simulink model "SCR_Buck_CL_17a"  (R2017b)
settings: Solver=FixedStepAuto  StartTime=0.0  StopTime=0.5  FixedStep=1e-6  MaxStep=1e-4  RelTol=1e-3
undefined symbols (not defined in the file): C
libraries: powerlib x16, simulink x5
settings Model: Creator=Suman Maiti  LastModifiedBy=Shuvam
settings DataIOCC: SaveFormat=StructureWithTime
settings OptimizationCC: LifeSpan=inf
settings DebuggingCC: AlgebraicLoopMsg=none  ArtificialAlgebraicLoopMsg=none  SFExecutionAtInitializationDiag=none
settings HardwareCC: ProdBitPerSizeT=32  ProdBitPerPtrDiffT=32  ProdWordSize=32  ProdHWDeviceType=Specified
settings CodeAppCC: StateflowObjectComments=on
settings SimscapeCC: SimscapeNormalizeSystem=off

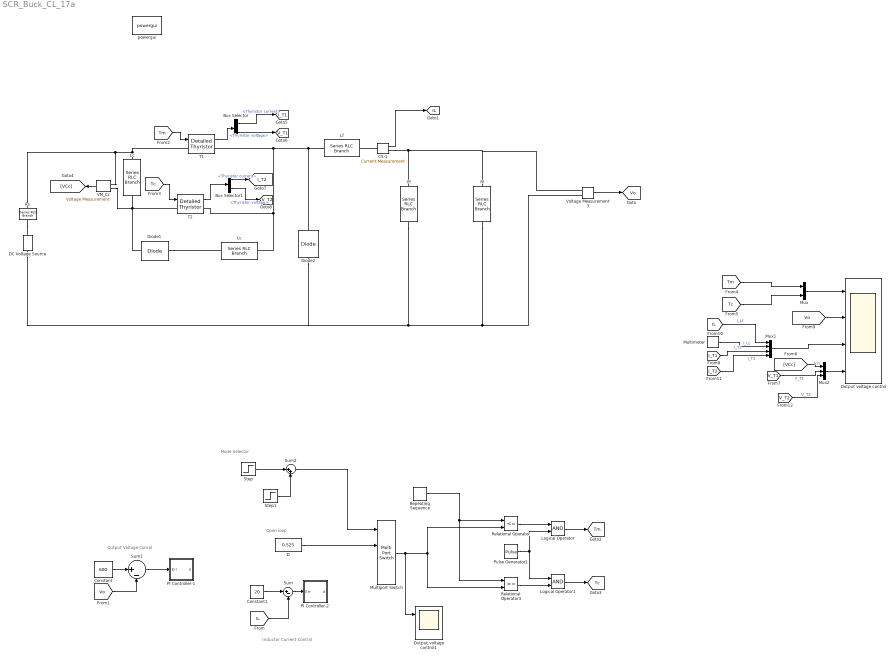
== system SCR_Buck_CL_17a ==
  note: Mode Selector
  note: Inductor Current Control
  note: Open loop
  note: Output Voltage Conrol
  Bus Selector : BusSelector  OutputSignals=Thyristor current,Thyristor voltage
  Bus Selector1 : BusSelector  OutputSignals=Thyristor current,Thyristor voltage
  CS-1 : powerlib/Measurements/Current Measurement  PhasorSimulation=off  OutputType=Complex  PSBequivalent=0
  Cc : powerlib/Elements/Series RLC Branch  LConnTagsString=__new0  RConnTagsString=__new0  BranchType=C  Resistance=0.00000001  Inductance=50e-3  SetiL0=off  InitialCurrent=0  Capacitance=0.2e-6  Setx0=on  InitialVoltage=1000  Measurements=None
  Cf : powerlib/Elements/Series RLC Branch  LConnTagsString=__new0  RConnTagsString=__new0  BranchType=C  Resistance=1  Inductance=15e-3  SetiL0=off  InitialCurrent=0  Capacitance=330e-6  Setx0=on  InitialVoltage=600  Measurements=None
  Constant : Constant  Value=600
  Constant1 : Constant  Value=20
  D : Constant  Value=0.525
  DC Voltage Source : powerlib/Electrical Sources/DC Voltage Source  Amplitude=1000  Measurements=None
  Diode1 : powerlib/Power Electronics/Diode  Ron=0.001  Lon=0  Vf=0  IC=0  UseSnubber=0  Rs=500  Cs=2e-9  Measurements=off
  Diode2 : powerlib/Power Electronics/Diode  Ron=0.001  Lon=0  Vf=0  IC=0  UseSnubber=0  Rs=500000  Cs=250e-9  Measurements=off
  Lc : powerlib/Elements/Series RLC Branch  LConnTagsString=__new0  RConnTagsString=__new0  BranchType=L  Resistance=1  Inductance=0.25e-3  SetiL0=off  InitialCurrent=0  Capacitance=C  Setx0=on  InitialVoltage=Vc  Measurements=Branch current
  Lf : powerlib/Elements/Series RLC Branch  LConnTagsString=__new0  RConnTagsString=__new0  BranchType=L  Resistance=1  Inductance=24e-3  SetiL0=off  InitialCurrent=0  Capacitance=C  Setx0=on  InitialVoltage=Vc  Measurements=None
  Logical Operator : Logic  AllPortsSameDT=off  OutDataTypeStr=boolean
  Logical Operator1 : Logic  AllPortsSameDT=off  OutDataTypeStr=boolean
  Multimeter : powerlib/Measurements/Multimeter  PhasorSimulation=off  OutputType=Complex  sel=1  L=1  Gain=1  yselected={'Ib: Lc'};  PSBOutputType=1  PSBequivalent=0  AxesSetting=[0,0.1,-100,100]  Display=0  SavedBlockNames=-11
  Multiport Switch : MultiPortSwitch  DataPortOrder=Zero-based contiguous
  Mux : Mux  Inputs=2
  Mux1 : Mux
  Mux2 : Mux  Inputs=3
  Output voltage control : Scope  NumInputPorts=4
  Output voltage control1 : Scope  NumInputPorts=2
  PI Controller-1 : Subsystem
  PI Controller-2 : Subsystem
  Pulse Generator1 : DiscretePulseGenerator  PulseType=Time based  Period=1/10000  PulseWidth=50
  Relational Operator : RelationalOperator  Operator=<=  OutDataTypeStr=boolean  RndMeth=Simplest
  Relational Operator3 : RelationalOperator  OutDataTypeStr=boolean  RndMeth=Simplest
  Repeating Sequence : simulink/Sources/Repeating Sequence  rep_seq_t=[0 0.002]  rep_seq_y=[0 1]
  Rl : powerlib/Elements/Series RLC Branch  LConnTagsString=__new0  RConnTagsString=__new0  BranchType=R  Resistance=30  Inductance=15e-3  SetiL0=off  InitialCurrent=0  Capacitance=330e-6  Setx0=on  InitialVoltage=Vc  Measurements=None
  Rs : powerlib/Elements/Series RLC Branch  LConnTagsString=__new0  RConnTagsString=__new0  BranchType=R  Resistance=0.00000001  Inductance=50e-3  SetiL0=off  InitialCurrent=0  Capacitance=4.7e-6  Setx0=on  InitialVoltage=200  Measurements=None
  Step : Step  SampleTime=0
  Step1 : Step  Time=2  SampleTime=0
  Sum : Sum  Inputs=|+-
  Sum1 : Sum  Inputs=|+-
  Sum2 : Sum  Inputs=|++
  T1 : powerlib/Power Electronics/Detailed Thyristor  Ron=0.000001  Lon=1e-6  Vf=0  IL=0.1  Tq=30e-6  IC=0  Rs=inf  Cs=0  Measurements=on
      settings: SourceProductName=Simscape Power Systems  SourceProductBaseCode=PS
  T2 : powerlib/Power Electronics/Detailed Thyristor  Ron=0.000001  Lon=1e-6  Vf=0  IL=0.1  Tq=30e-6  IC=0  Rs=inf  Cs=0  Measurements=on
      settings: SourceProductName=Simscape Power Systems  SourceProductBaseCode=PS
  VM_Cc : powerlib/Measurements/Voltage Measurement  PhasorSimulation=off  OutputType=Complex  PSBequivalent=0
  Voltage Measurement3 : powerlib/Measurements/Voltage Measurement  PhasorSimulation=off  OutputType=Complex  PSBequivalent=0
  powergui : powerlib/powergui  Priority=1  SimulationMode=Discrete  SampleTime=1e-6  frequency=60  Iterations=50  frequencyindice=0  Pbase=100e6  ErrMax=1e-4  UnitsV=kV  UnitsW=MW  buscounter=0  FunctionMessages=off  echomessages=off  EnableUseOfTLC=off  CurrentSourceSwitches=off  DisableSnubberDevices=off  DisableRonSwitches=off  DisableVfSwitches=off  DisplayEquations=off  SolverType=Tustin/Backward Euler (TBE)  Interpol=off  ExternalGateDelay=off  methode=off  Ts=100  x0status=blocks  SPID=off  SwTol=0  HookPort=off  RestoreLinks=warning  ResistiveCurrentMeasurement=off  Frange=[0:2:500]  Ylog=off  Xlog=on  ShowGrid=off  save=off  variable=ZData  structure=ScopeData1  ZoomFFT=off  StartTime=1.45  cycles=2  DisplayStyle=1  fundamental=50  FreqAxis=off  MaxFrequency=2000  frequencyindicesteady=1  RmsSteady=1  display=off
  tag scope: IL=global, I_T1=global, I_T2=global, Tc=global, Tm=global, V_T1=global, V_T2=global, Vo=global
  wires:
  Voltage Measurement3/1 -> [Vo]
  [Tc] -> T2/1
  CS-1/1 -> [IL]
  [Tm] -> T1/1
  [IL] -> Sum/2
  Relational Operator/1 -> Logical Operator/1
  Pulse Generator1/1 -> Logical Operator1/1, Logical Operator/2
  Repeating Sequence/1 -> Relational Operator/1, Relational Operator3/1
  Relational Operator3/1 -> Logical Operator1/2
  Logical Operator/1 -> [Tm]
  Logical Operator1/1 -> [Tc]
  [Vo] -> Sum1/2
  Constant/1 -> Sum1/1
  Sum/1 -> PI Controller-2/1(Err)
  Constant1/1 -> Sum/1
  Step/1 -> Sum2/1
  Step1/1 -> Sum2/2
  Sum2/1 -> Multiport Switch/1
  [Vo] -> Output voltage control/2
  Mux1/1 -> Output voltage control/3
  Mux/1 -> Output voltage control/1
  [Tm] -> Mux/1
  [Tc] -> Mux/2
  [VCc] -> Mux2/1  "Vcc"
  VM_Cc/1 -> [VCc]
  Sum1/1 -> PI Controller-1/1(Err)
  Multimeter/1 -> Mux1/2  "I_Lc"
  [IL] -> Mux1/1  "I_Lf"
  D/1 -> Multiport Switch/2
  T1/1 -> Bus Selector/1
  Bus Selector/1 -> [I_T1]  "<Thyristor current>"
  Bus Selector/2 -> [V_T1]  "<Thyristor voltage>"
  T2/1 -> Bus Selector1/1
  Bus Selector1/1 -> [I_T2]  "<Thyristor current>"
  Bus Selector1/2 -> [V_T2]  "<Thyristor voltage>"
  [I_T1] -> Mux1/3  "I_T1"
  [I_T2] -> Mux1/4  "I_T2"
  [V_T1] -> Mux2/2  "V_T1"
  [V_T2] -> Mux2/3  "V_T2"
  Mux2/1 -> Output voltage control/4
  Multiport Switch/1 -> Output voltage control1/1, Relational Operator3/2, Relational Operator/2
  connections:
  VM_Cc/LConn2 -- Diode1/RConn1 -- T2/LConn1 -- Cc/RConn1
  Diode2/RConn1 -- T1/RConn1 -- T2/RConn1 -- Lc/LConn1 -- Lf/RConn1
  Voltage Measurement3/LConn1 -- Rl/LConn1 -- Cf/LConn1 -- CS-1/RConn1
  Rl/RConn1 -- Diode2/LConn1 -- DC Voltage Source/LConn1 -- Cf/RConn1 -- Voltage Measurement3/LConn2
  Diode1/LConn1 -- Lc/RConn1
  CS-1/LConn1 -- Lf/LConn1
  Rs/RConn1 -- DC Voltage Source/RConn1
  Cc/LConn1 -- T1/LConn1 -- VM_Cc/LConn1 -- Rs/LConn1

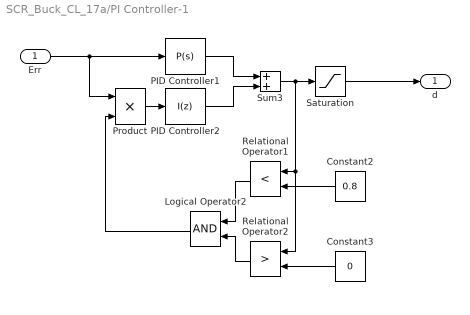
== system SCR_Buck_CL_17a/PI Controller-1 ==
  Err : Inport
  Constant2 : Constant  Value=0.8
  Constant3 : Constant  Value=0
  Logical Operator2 : Logic  AllPortsSameDT=off  OutDataTypeStr=boolean
  PID Controller1 : simulink/Continuous/PID Controller  Controller=P  TimeDomain=Continuous-time  SampleTime=-1  IntegratorMethod=Forward Euler  FilterMethod=Forward Euler  Form=Parallel  UseFilter=on  ControllerParametersSource=internal  P=1/(2.25*800)  I=23.22*1/(2.25*800)  D=0  N=100  InitialConditionSource=internal  InitialConditionForIntegrator=0  InitialConditionForFilter=0  ExternalReset=none  LimitOutput=off  UpperSaturationLimit=0.8  LowerSaturationLimit=0.2  LinearizeAsGain=on  AntiWindupMode=none  Kb=1  TrackingMode=off  Kt=1  PParamMin=[]  PParamMax=[]  IParamMin=[]  IParamMax=[]  DParamMin=[]  DParamMax=[]  NParamMin=[]  NParamMax=[]  KbParamMin=[]  KbParamMax=[]  KtParamMin=[]  KtParamMax=[]  POutMin=[]  POutMax=[]  IOutMin=[]  IOutMax=[]  DOutMin=[]  DOutMax=[]  NOutMin=[]  NOutMax=[]  KbOutMin=[]  KbOutMax=[]  KtOutMin=[]  KtOutMax=[]  IntegratorOutMin=[]  IntegratorOutMax=[]  FilterOutMin=[]  FilterOutMax=[]  SumOutMin=[]  SumOutMax=[]  SumI1OutMin=[]  SumI1OutMax=[]  SumI2OutMin=[]  SumI2OutMax=[]  SumI3OutMin=[]  SumI3OutMax=[]  SumDOutMin=[]  SumDOutMax=[]  SaturationOutMin=[]  SaturationOutMax=[]  IntegratorContinuousStateAttributes=''  IntegratorStateMustResolveToSignalObject=off  IntegratorRTWStateStorageClass=Auto  FilterContinuousStateAttributes=''  FilterStateMustResolveToSignalObject=off  FilterRTWStateStorageClass=Auto  DifferentiatorICPrevScaledInput=0  DifferentiatorOutMin=[]  DifferentiatorOutMax=[]  InitialConditionSetting=State (most efficient)  FilterDiffOutCoefMin=[]  FilterDiffOutCoefMax=[]  SumDenOutMin=[]  SumDenOutMax=[]  SumNumOutMin=[]  SumNumOutMax=[]  ReciprocalOutMin=[]  ReciprocalOutMax=[]  DivideOutMin=[]  DivideOutMax=[]  TunerSelectOption=Transfer Function Based (PID Tuner App)
  PID Controller2 : simulink/Continuous/PID Controller  Controller=I  TimeDomain=Discrete-time  SampleTime=-1  IntegratorMethod=Forward Euler  FilterMethod=Forward Euler  Form=Parallel  UseFilter=on  ControllerParametersSource=internal  P=1/(2.25*800)  I=23.22*1/(2.25*800)  D=0  N=100  InitialConditionSource=internal  InitialConditionForIntegrator=0  InitialConditionForFilter=0  ExternalReset=none  LimitOutput=off  UpperSaturationLimit=0.8  LowerSaturationLimit=0.2  LinearizeAsGain=on  AntiWindupMode=none  Kb=1  TrackingMode=off  Kt=1  PParamMin=[]  PParamMax=[]  IParamMin=[]  IParamMax=[]  DParamMin=[]  DParamMax=[]  NParamMin=[]  NParamMax=[]  KbParamMin=[]  KbParamMax=[]  KtParamMin=[]  KtParamMax=[]  POutMin=[]  POutMax=[]  IOutMin=[]  IOutMax=[]  DOutMin=[]  DOutMax=[]  NOutMin=[]  NOutMax=[]  KbOutMin=[]  KbOutMax=[]  KtOutMin=[]  KtOutMax=[]  IntegratorOutMin=[]  IntegratorOutMax=[]  FilterOutMin=[]  FilterOutMax=[]  SumOutMin=[]  SumOutMax=[]  SumI1OutMin=[]  SumI1OutMax=[]  SumI2OutMin=[]  SumI2OutMax=[]  SumI3OutMin=[]  SumI3OutMax=[]  SumDOutMin=[]  SumDOutMax=[]  SaturationOutMin=[]  SaturationOutMax=[]  IntegratorContinuousStateAttributes=''  IntegratorStateMustResolveToSignalObject=off  IntegratorRTWStateStorageClass=Auto  FilterContinuousStateAttributes=''  FilterStateMustResolveToSignalObject=off  FilterRTWStateStorageClass=Auto  DifferentiatorICPrevScaledInput=0  DifferentiatorOutMin=[]  DifferentiatorOutMax=[]  InitialConditionSetting=State (most efficient)  FilterDiffOutCoefMin=[]  FilterDiffOutCoefMax=[]  SumDenOutMin=[]  SumDenOutMax=[]  SumNumOutMin=[]  SumNumOutMax=[]  ReciprocalOutMin=[]  ReciprocalOutMax=[]  DivideOutMin=[]  DivideOutMax=[]  TunerSelectOption=Transfer Function Based (PID Tuner App)
  Product : Product
  Relational Operator1 : RelationalOperator  Operator=<  OutDataTypeStr=boolean  RndMeth=Simplest
  Relational Operator2 : RelationalOperator  Operator=>  OutDataTypeStr=boolean  RndMeth=Simplest
  Saturation : Saturate  UpperLimit=0.8  LowerLimit=0.1
  Sum3 : Sum
  d : Outport
  wires:
  Err/1 -> Product/1, PID Controller1/1
  Saturation/1 -> d/1
  PID Controller2/1 -> Sum3/2
  Product/1 -> PID Controller2/1
  PID Controller1/1 -> Sum3/1
  Constant3/1 -> Relational Operator2/2
  Logical Operator2/1 -> Product/2
  Relational Operator1/1 -> Logical Operator2/1
  Sum3/1 -> Saturation/1, Relational Operator2/1, Relational Operator1/1
  Relational Operator2/1 -> Logical Operator2/2
  Constant2/1 -> Relational Operator1/2

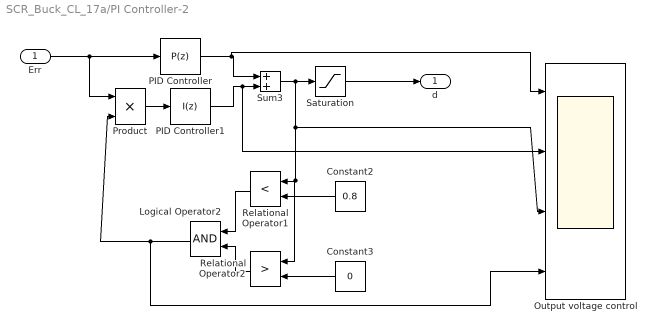
== system SCR_Buck_CL_17a/PI Controller-2 ==
  Err : Inport
  Constant2 : Constant  Value=0.8
  Constant3 : Constant  Value=0
  Logical Operator2 : Logic  AllPortsSameDT=off  OutDataTypeStr=boolean
  Output voltage control : Scope  NumInputPorts=4
  PID Controller : simulink/Continuous/PID Controller  Controller=P  TimeDomain=Discrete-time  SampleTime=-1  IntegratorMethod=Forward Euler  FilterMethod=Forward Euler  Form=Parallel  UseFilter=on  ControllerParametersSource=internal  P=4.8474/800  I=52.47*4.8474/800  D=0  N=100  InitialConditionSource=internal  InitialConditionForIntegrator=0  InitialConditionForFilter=0  ExternalReset=none  LimitOutput=off  UpperSaturationLimit=0.8  LowerSaturationLimit=0.2  LinearizeAsGain=on  AntiWindupMode=none  Kb=1  TrackingMode=off  Kt=1  PParamMin=[]  PParamMax=[]  IParamMin=[]  IParamMax=[]  DParamMin=[]  DParamMax=[]  NParamMin=[]  NParamMax=[]  KbParamMin=[]  KbParamMax=[]  KtParamMin=[]  KtParamMax=[]  POutMin=[]  POutMax=[]  IOutMin=[]  IOutMax=[]  DOutMin=[]  DOutMax=[]  NOutMin=[]  NOutMax=[]  KbOutMin=[]  KbOutMax=[]  KtOutMin=[]  KtOutMax=[]  IntegratorOutMin=[]  IntegratorOutMax=[]  FilterOutMin=[]  FilterOutMax=[]  SumOutMin=[]  SumOutMax=[]  SumI1OutMin=[]  SumI1OutMax=[]  SumI2OutMin=[]  SumI2OutMax=[]  SumI3OutMin=[]  SumI3OutMax=[]  SumDOutMin=[]  SumDOutMax=[]  SaturationOutMin=[]  SaturationOutMax=[]  IntegratorContinuousStateAttributes=''  IntegratorStateMustResolveToSignalObject=off  IntegratorRTWStateStorageClass=Auto  FilterContinuousStateAttributes=''  FilterStateMustResolveToSignalObject=off  FilterRTWStateStorageClass=Auto  DifferentiatorICPrevScaledInput=0  DifferentiatorOutMin=[]  DifferentiatorOutMax=[]  InitialConditionSetting=State (most efficient)  FilterDiffOutCoefMin=[]  FilterDiffOutCoefMax=[]  SumDenOutMin=[]  SumDenOutMax=[]  SumNumOutMin=[]  SumNumOutMax=[]  ReciprocalOutMin=[]  ReciprocalOutMax=[]  DivideOutMin=[]  DivideOutMax=[]  TunerSelectOption=Transfer Function Based (PID Tuner App)
  PID Controller1 : simulink/Continuous/PID Controller  Controller=I  TimeDomain=Discrete-time  SampleTime=-1  IntegratorMethod=Forward Euler  FilterMethod=Forward Euler  Form=Parallel  UseFilter=on  ControllerParametersSource=internal  P=4.8474/800  I=52.47*4.8474/800  D=0  N=100  InitialConditionSource=internal  InitialConditionForIntegrator=0  InitialConditionForFilter=0  ExternalReset=none  LimitOutput=off  UpperSaturationLimit=0.8  LowerSaturationLimit=0.2  LinearizeAsGain=on  AntiWindupMode=none  Kb=1  TrackingMode=off  Kt=1  PParamMin=[]  PParamMax=[]  IParamMin=[]  IParamMax=[]  DParamMin=[]  DParamMax=[]  NParamMin=[]  NParamMax=[]  KbParamMin=[]  KbParamMax=[]  KtParamMin=[]  KtParamMax=[]  POutMin=[]  POutMax=[]  IOutMin=[]  IOutMax=[]  DOutMin=[]  DOutMax=[]  NOutMin=[]  NOutMax=[]  KbOutMin=[]  KbOutMax=[]  KtOutMin=[]  KtOutMax=[]  IntegratorOutMin=[]  IntegratorOutMax=[]  FilterOutMin=[]  FilterOutMax=[]  SumOutMin=[]  SumOutMax=[]  SumI1OutMin=[]  SumI1OutMax=[]  SumI2OutMin=[]  SumI2OutMax=[]  SumI3OutMin=[]  SumI3OutMax=[]  SumDOutMin=[]  SumDOutMax=[]  SaturationOutMin=[]  SaturationOutMax=[]  IntegratorContinuousStateAttributes=''  IntegratorStateMustResolveToSignalObject=off  IntegratorRTWStateStorageClass=Auto  FilterContinuousStateAttributes=''  FilterStateMustResolveToSignalObject=off  FilterRTWStateStorageClass=Auto  DifferentiatorICPrevScaledInput=0  DifferentiatorOutMin=[]  DifferentiatorOutMax=[]  InitialConditionSetting=State (most efficient)  FilterDiffOutCoefMin=[]  FilterDiffOutCoefMax=[]  SumDenOutMin=[]  SumDenOutMax=[]  SumNumOutMin=[]  SumNumOutMax=[]  ReciprocalOutMin=[]  ReciprocalOutMax=[]  DivideOutMin=[]  DivideOutMax=[]  TunerSelectOption=Transfer Function Based (PID Tuner App)
  Product : Product
  Relational Operator1 : RelationalOperator  Operator=<  OutDataTypeStr=boolean  RndMeth=Simplest
  Relational Operator2 : RelationalOperator  Operator=>  OutDataTypeStr=boolean  RndMeth=Simplest
  Saturation : Saturate  UpperLimit=0.8  LowerLimit=0.1
  Sum3 : Sum
  d : Outport
  wires:
  Logical Operator2/1 -> Output voltage control/4, Product/2
  Err/1 -> PID Controller/1, Product/1
  Constant2/1 -> Relational Operator1/2
  Relational Operator1/1 -> Logical Operator2/1
  Product/1 -> PID Controller1/1
  Saturation/1 -> d/1
  Constant3/1 -> Relational Operator2/2
  Sum3/1 -> Output voltage control/3, Relational Operator2/1, Relational Operator1/1, Saturation/1
  Relational Operator2/1 -> Logical Operator2/2
  PID Controller/1 -> Output voltage control/1, Sum3/1
  PID Controller1/1 -> Output voltage control/2, Sum3/2
